simulink model "Open_and_Closed_Loop_Systems_without_Controllers"  (R2024b)
settings: Solver=VariableStepAuto  StartTime=0.0  StopTime=10.0  RelTol=1e-3
libraries: simulink x4
settings Model: Creator=LEGION  LastModifiedBy=LEGION

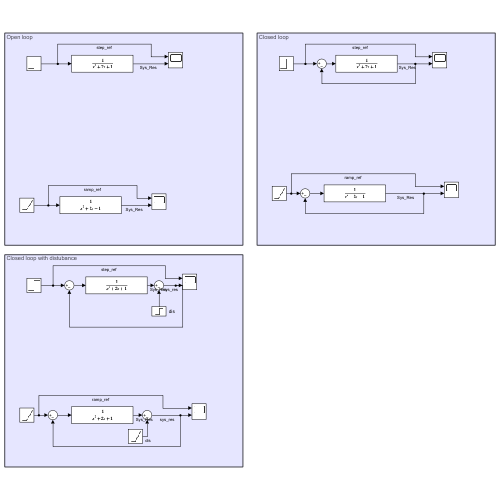
[thumbnail: Simulink's stored preview of the top-level diagram]
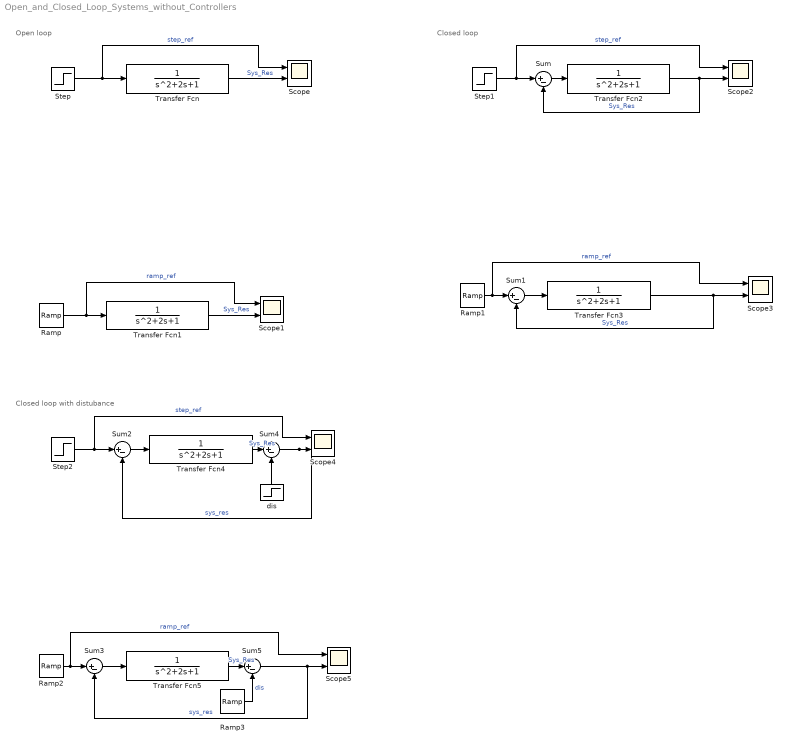
== system Open_and_Closed_Loop_Systems_without_Controllers ==
  note: Open loop
  note: Closed loop
  note: Closed loop with distubance
  Ramp : simulink/Sources/Ramp  slope=1  start=0  InitialOutput=0
  Ramp1 : simulink/Sources/Ramp  slope=1  start=0  InitialOutput=0
  Ramp2 : simulink/Sources/Ramp  slope=1  start=0  InitialOutput=0
  Ramp3 : simulink/Sources/Ramp  slope=0.5  start=0  InitialOutput=0
  Scope{,1..5} (6 alike) : Scope  NumInputPorts=2
  Step : Step  SampleTime=0
  Step1 : Step  SampleTime=0
  Step2 : Step  SampleTime=0
  Sum{,1..5} (6 alike) : Sum  Inputs=|+-
  Transfer Fcn{,1..5} (6 alike) : TransferFcn
  dis : Step  Time=4  After=0.35  SampleTime=0
  wires:
  Step/1 -> Scope/1, Transfer Fcn/1  "step_ref"
  Ramp/1 -> Scope1/1, Transfer Fcn1/1  "ramp_ref"
  Transfer Fcn/1 -> Scope/2  "Sys_Res"
  Transfer Fcn1/1 -> Scope1/2  "Sys_Res"
  Transfer Fcn3/1 -> Sum1/2, Scope3/2  "Sys_Res"
  Step1/1 -> Sum/1, Scope2/1  "step_ref"
  Ramp1/1 -> Sum1/1, Scope3/1  "ramp_ref"
  Transfer Fcn2/1 -> Scope2/2, Sum/2  "Sys_Res"
  Sum/1 -> Transfer Fcn2/1
  Sum1/1 -> Transfer Fcn3/1
  Sum3/1 -> Transfer Fcn5/1
  Sum2/1 -> Transfer Fcn4/1
  Ramp2/1 -> Sum3/1, Scope5/1  "ramp_ref"
  Step2/1 -> Sum2/1, Scope4/1  "step_ref"
  Transfer Fcn4/1 -> Sum4/1  "Sys_Res"
  Sum4/1 -> Scope4/2, Sum2/2  "sys_res"
  dis/1 -> Sum4/2
  Transfer Fcn5/1 -> Sum5/1  "Sys_Res"
  Sum5/1 -> Sum3/2, Scope5/2  "sys_res"
  Ramp3/1 -> Sum5/2  "dis"
